simulink model "equivalence_sliding_mode"  (R2019b)
settings: Solver=VariableStepAuto  StartTime=0.0  StopTime=20  RelTol=1e-3
libraries: fuzblock x1
settings Model: Creator=Alien  LastModifiedBy=Alien
settings SolverCC: ZeroCrossAlgorithm=Adaptive
settings DebuggingCC: IgnoredZcDiagnostic=none

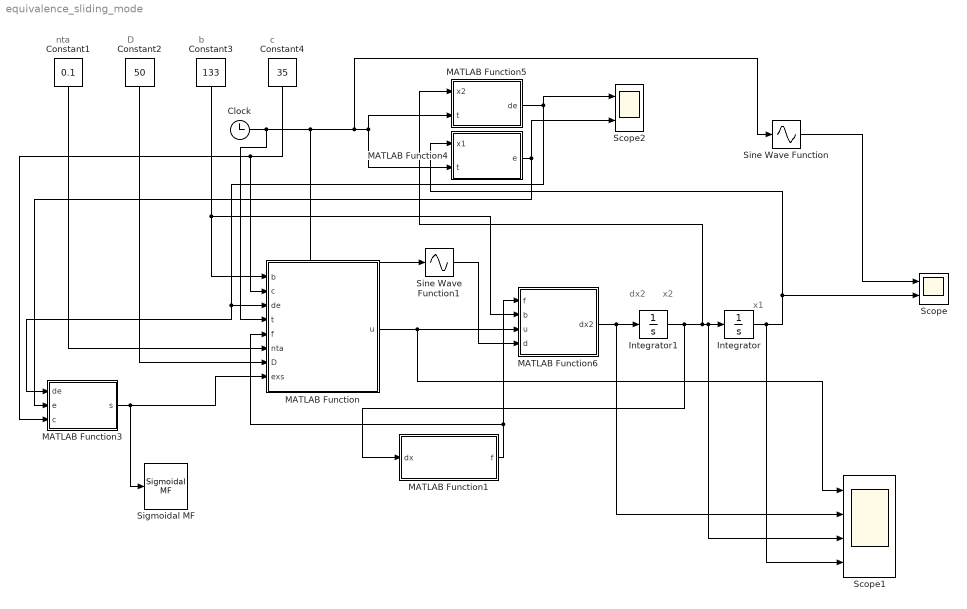
== system equivalence_sliding_mode ==
  note: c
  note: b
  note: D
  note: nta
  note: dx2
  note: x2
  note: x1
  Clock : Clock
  Constant1 : Constant  Value=0.1
  Constant2 : Constant  Value=50
  Constant3 : Constant  Value=133
  Constant4 : Constant  Value=35
  Integrator : Integrator  InitialCondition=0.5
  Integrator1 : Integrator  InitialCondition=2
  MATLAB Function : MATLAB Function  TreatAsAtomicUnit=on
  MATLAB Function1 : MATLAB Function  TreatAsAtomicUnit=on
  MATLAB Function3 : MATLAB Function  TreatAsAtomicUnit=on
  MATLAB Function4 : MATLAB Function  TreatAsAtomicUnit=on
  MATLAB Function5 : MATLAB Function  TreatAsAtomicUnit=on
  MATLAB Function6 : MATLAB Function  TreatAsAtomicUnit=on
  Scope : Scope  NumInputPorts=2
  Scope1 : Scope  NumInputPorts=4
  Scope2 : Scope  NumInputPorts=2
  Sigmoidal MF : fuzblock/Membership  Functions/Sigmoidal MF  a=1  c=0
      settings: SourceProductName=Fuzzy Logic Toolbox  SourceProductBaseCode=FL
  Sine Wave Function : Sin  TimeSource=Use external signal  Frequency=2*pi  SampleTime=0
  Sine Wave Function1 : Sin  TimeSource=Use external signal  Amplitude=50  SampleTime=0
  wires:
  Integrator1/1 -> MATLAB Function1/1(dx), MATLAB Function5/1(x2), Scope1/3, Integrator/1
  MATLAB Function6/1(dx2) -> Scope1/2, Integrator1/1
  MATLAB Function1/1(f) -> MATLAB Function6/1(f), MATLAB Function/5(f)
  MATLAB Function5/1(de) -> MATLAB Function3/1(de), MATLAB Function/3(de), Scope2/1
  Integrator/1 -> Scope1/4, Scope/2, MATLAB Function4/1(x1)
  MATLAB Function4/1(e) -> MATLAB Function3/2(e), Scope2/2
  Clock/1 -> MATLAB Function/4(t), Sine Wave Function1/1, Sine Wave Function/1, MATLAB Function4/2(t), MATLAB Function5/2(t)
  Sine Wave Function/1 -> Scope/1
  MATLAB Function/1(u) -> Scope1/1, MATLAB Function6/3(u)
  Sine Wave Function1/1 -> MATLAB Function6/4(d)
  Constant4/1 -> MATLAB Function3/3(c), MATLAB Function/2(c)
  Constant3/1 -> MATLAB Function6/2(b), MATLAB Function/1(b)
  MATLAB Function3/1(s) -> MATLAB Function/8(exs), Sigmoidal MF/1
  Constant2/1 -> MATLAB Function/7(D)
  Constant1/1 -> MATLAB Function/6(nta)

== matlab function equivalence_sliding_mode/MATLAB Function1 ==
  data: dx input; f output
function f = fcn(dx)
f = -25 * dx;

== matlab function equivalence_sliding_mode/MATLAB Function ==
  data: b input; c input; de input; t input; u output; f input; nta input; D input; exs input
function u = fcn(b, c, de, t, f, nta, D, exs)
ddxd = -((2*pi)^2)*sin(2*pi*t);
u = 1/b*(ddxd - f + c * de + (nta + D) * sign(exs));

== matlab function equivalence_sliding_mode/MATLAB Function3 ==
  data: de input; s output; e input; c input
function s = fcn(de, e, c)
s = de + c*e;

== matlab function equivalence_sliding_mode/MATLAB Function4 ==
  data: x1 input; e output; t input
function e = fcn(x1, t)
e = sin(2*pi*t) - x1;

== matlab function equivalence_sliding_mode/MATLAB Function5 ==
  data: x2 input; de output; t input
function de = fcn(x2, t)
de = 2*pi*cos(2*pi*t) - x2;

== matlab function equivalence_sliding_mode/MATLAB Function6 ==
  data: f input; b input; u input; dx2 output; d input
function dx2 = fcn(f, b, u, d)
dx2 = f + b*u + d;
